simulink model "model"  (R2021a)
settings: Solver=FixedStepAuto  StartTime=0.0  StopTime=2  FixedStep=step  RelTol=1e-3
undefined symbols (not defined in the file or in its folder): qc
libraries: roblocks x7, simulink x2
settings Model: Creator=ohvic  LastModifiedBy=ohvic

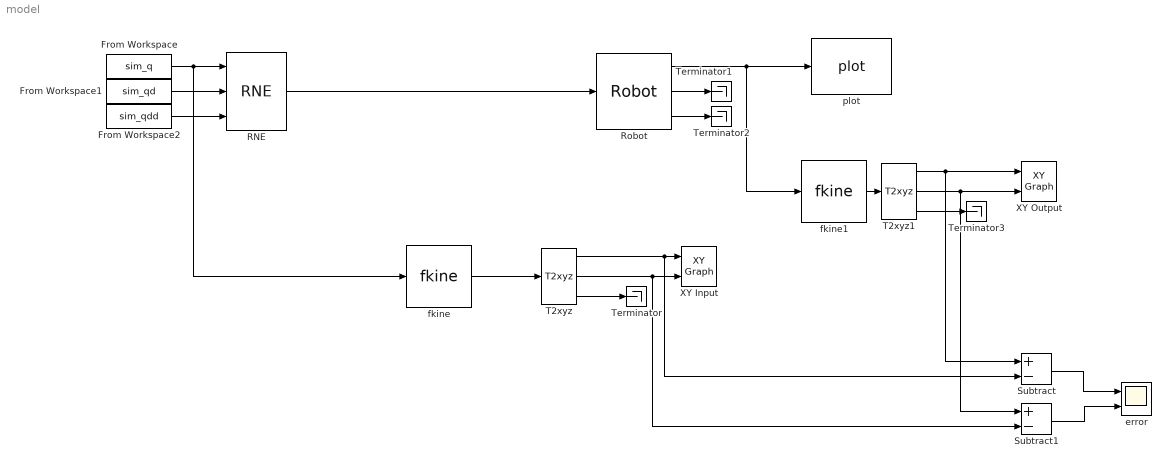
== system model ==
  From Workspace : FromWorkspace  VariableName=sim_q  SampleTime=-1
  From Workspace1 : FromWorkspace  VariableName=sim_qd  SampleTime=-1
  From Workspace2 : FromWorkspace  VariableName=sim_qdd  SampleTime=-1
  RNE : roblocks/Arm/RNE  robot=robot  grav=[0 0 9.81]
  Robot : roblocks/Arm/Robot  robot=robot  q0=qc(1,:)
  Subtract : Sum  Inputs=+-
  Subtract1 : Sum  Inputs=+-
  T2xyz : roblocks/Toolbox/T2xyz
  T2xyz1 : roblocks/Toolbox/T2xyz
  Terminator{,1..3} (4 alike) : Terminator
  XY Input : simulink/Sinks/XY Graph  xmin=-2  xmax=2  ymin=-2  ymax=2  st=-1
  XY Output : simulink/Sinks/XY Graph  xmin=-2  xmax=2  ymin=-2  ymax=2  st=-1
  error : Scope  NumInputPorts=2
  fkine : roblocks/Arm/fkine  robot=robot
  fkine1 : roblocks/Arm/fkine  robot=robot
  plot : roblocks/Arm/plot  robot=robot  fps=5  holdplot=on
  wires:
  From Workspace/1 -> RNE/1, fkine/1
  From Workspace1/1 -> RNE/2
  From Workspace2/1 -> RNE/3
  Robot/1 -> fkine1/1, plot/1
  fkine/1 -> T2xyz/1
  T2xyz/3 -> Terminator/1
  T2xyz/2 -> Subtract1/2, XY Input/2
  T2xyz/1 -> Subtract/2, XY Input/1
  Robot/2 -> Terminator1/1
  Robot/3 -> Terminator2/1
  fkine1/1 -> T2xyz1/1
  T2xyz1/3 -> Terminator3/1
  T2xyz1/1 -> Subtract/1, XY Output/1
  T2xyz1/2 -> Subtract1/1, XY Output/2
  RNE/1 -> Robot/1
  Subtract/1 -> error/1
  Subtract1/1 -> error/2
